simulink model "ModelEnv_Test_Erreur_tracker_v2"  (R2020b)
settings: Solver=VariableStepAuto  StartTime=0.0  StopTime=24  RelTol=1e-3
undefined symbols (not defined in the file): alpha, Atz, Bd, Bh, gama, theta, Ts, Tz_init
libraries: dspsrcs4 x2
settings Model: Creator=masdoua1  LastModifiedBy=masdoua1

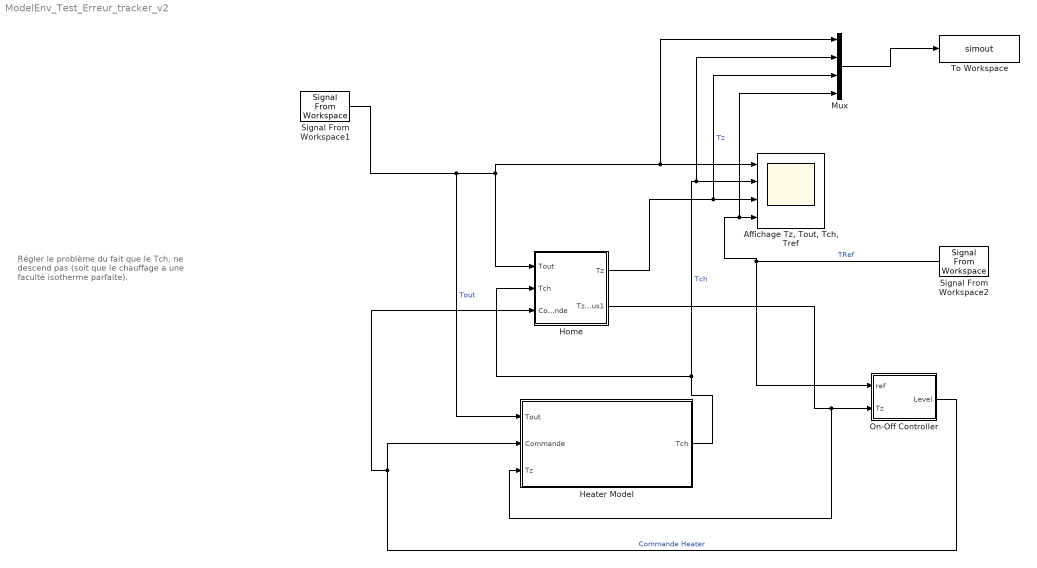
== system ModelEnv_Test_Erreur_tracker_v2 ==
  note: Régler le problème du fait que le Tch, ne descend pas (soit que le chauffage a une faculté isotherme parfaite).
  "Affichage Tz, Tout, Tch, Tref" : Scope  NumInputPorts=4
  Heater Model : Subsystem
  Home : Subsystem
  Mux : Mux
      settings: DisplayOption=signals
  On-Off Controller : MATLAB Function  TreatAsAtomicUnit=on
  Signal From Workspace1 : dspsrcs4/Signal From Workspace  X=Tout  Ts=1  nsamps=1  OutputAfterFinalValue=Setting to zero  ignoreOrWarnInputAndFrameLengths=off  OutputFrames=off
  Signal From Workspace2 : dspsrcs4/Signal From Workspace  X=Ref  Ts=1  nsamps=1  OutputAfterFinalValue=Setting to zero  ignoreOrWarnInputAndFrameLengths=off  OutputFrames=off
  To Workspace : ToWorkspace  VariableName=simout  SaveFormat=Timeseries  SampleTime=-1
  wires:
  On-Off Controller/1(Level) -> Heater Model/2(Commande), Home/3(Commande)  "Commande Heater"
  Signal From Workspace2/1 -> On-Off Controller/1(ref), Mux/4, "Affichage Tz, Tout, Tch, Tref"/4  "TRef"
  Heater Model/1(Tch) -> Mux/2, "Affichage Tz, Tout, Tch, Tref"/2, Home/2(Tch)  "Tch"
  Signal From Workspace1/1 -> Heater Model/1(Tout), Home/1(Tout), Mux/1, "Affichage Tz, Tout, Tch, Tref"/1  "Tout"
  Home/2(Tz_minus1) -> Heater Model/3(Tz), On-Off Controller/2(Tz)
  Home/1(Tz) -> Mux/3, "Affichage Tz, Tout, Tch, Tref"/3  "Tz"
  Mux/1 -> To Workspace/1

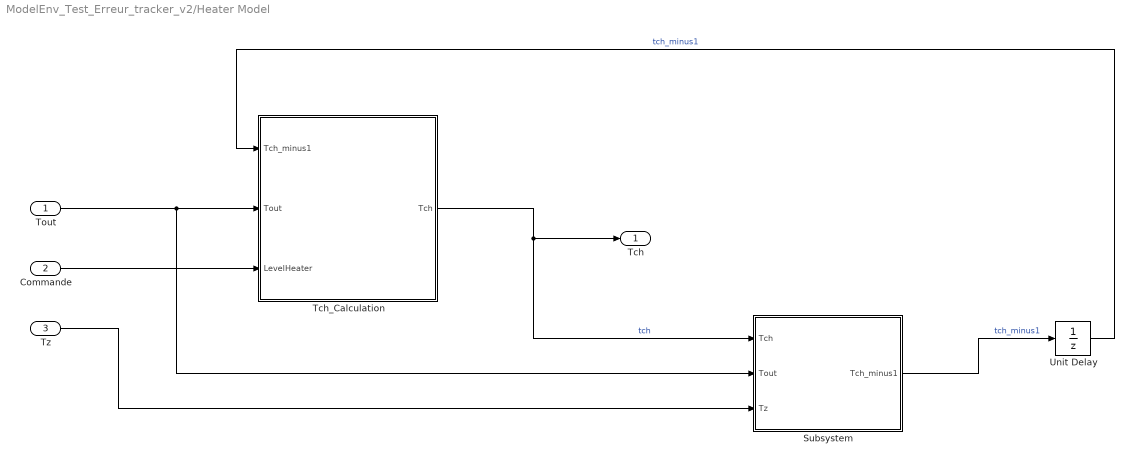
== system ModelEnv_Test_Erreur_tracker_v2/Heater Model ==
  Tout : Inport
  Commande : Inport  Port=2
  Tz : Inport  Port=3
  Subsystem : Subsystem
  Tch_Calculation : MATLAB Function  TreatAsAtomicUnit=on
  Unit Delay : UnitDelay  SampleTime=-1  HasFrameUpgradeWarning=on
  Tch : Outport
  wires:
  Tout/1 -> Subsystem/2(Tout), Tch_Calculation/2(Tout)
  Commande/1 -> Tch_Calculation/3(LevelHeater)
  Tch_Calculation/1(Tch) -> Subsystem/1(Tch), Tch/1  "tch"
  Unit Delay/1 -> Tch_Calculation/1(Tch_minus1)  "tch_minus1"
  Tz/1 -> Subsystem/3(Tz)
  Subsystem/1(Tch_minus1) -> Unit Delay/1  "tch_minus1"

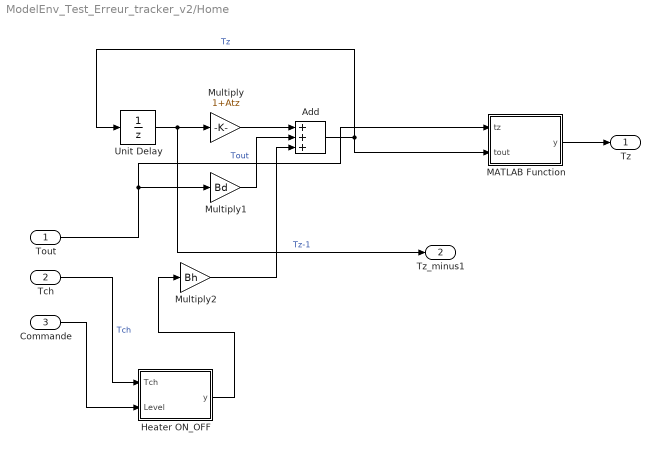
== system ModelEnv_Test_Erreur_tracker_v2/Home ==
  Tout : Inport
  Tch : Inport  Port=2
  Commande : Inport  Port=3
  Add : Sum  Inputs=+++
  Heater ON_OFF : MATLAB Function  TreatAsAtomicUnit=on
  MATLAB Function : MATLAB Function  TreatAsAtomicUnit=on
  Multiply : Gain  Gain=1+Atz
  Multiply1 : Gain  Gain=Bd
  Multiply2 : Gain  Gain=Bh
  Unit Delay : UnitDelay  InitialCondition=Tz_init  SampleTime=Ts  HasFrameUpgradeWarning=on
  Tz : Outport
  Tz_minus1 : Outport  Port=2
  wires:
  Multiply/1 -> Add/1
  Unit Delay/1 -> Tz_minus1/1, Multiply/1  "Tz-1"
  Tout/1 -> MATLAB Function/1(tz), Multiply1/1  "Tout"
  Multiply1/1 -> Add/2
  Add/1 -> Unit Delay/1, MATLAB Function/2(tout)  "Tz"
  Multiply2/1 -> Add/3
  Commande/1 -> Heater ON_OFF/2(Level)
  Tch/1 -> Heater ON_OFF/1(Tch)  "Tch"
  Heater ON_OFF/1(y) -> Multiply2/1
  MATLAB Function/1(y) -> Tz/1

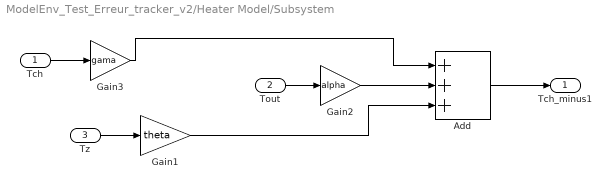
== system ModelEnv_Test_Erreur_tracker_v2/Heater Model/Subsystem ==
  Tch : Inport
  Tout : Inport  Port=2
  Tz : Inport  Port=3
  Add : Sum  Inputs=+++
  Gain1 : Gain  Gain=theta
  Gain2 : Gain  Gain=alpha
  Gain3 : Gain  Gain=gama
  Tch_minus1 : Outport
  wires:
  Add/1 -> Tch_minus1/1
  Gain1/1 -> Add/3
  Tz/1 -> Gain1/1
  Tout/1 -> Gain2/1
  Gain2/1 -> Add/2
  Tch/1 -> Gain3/1
  Gain3/1 -> Add/1

== matlab function ModelEnv_Test_Erreur_tracker_v2/Heater Model/Tch_Calculation ==
  data: Tch_minus1 input; Tout input; LevelHeater input; Tch output
function Tch = fcn(Tch_minus1, Tout, LevelHeater)
    
    if Tout > Tch_minus1
        Tch_minus1 = Tout+0.2; 
    end
    
    Tch = Tch_minus1 + LevelHeater;

== matlab function ModelEnv_Test_Erreur_tracker_v2/On-Off Controller ==
  data: ref input; Tz input; Level output
function Level= fcn(ref, Tz)

err = ref - Tz;
if err > 0
    Level = 5;
else
    Level = 0;
end
    
end

== matlab function ModelEnv_Test_Erreur_tracker_v2/Home/Heater ON_OFF ==
  data: Tch input; Level input; y output
function y = fcn(Tch, Level)
y = Tch;
if Level ==0
        y = 0;
end

== matlab function ModelEnv_Test_Erreur_tracker_v2/Home/MATLAB Function ==
  data: tz input; tout input; y output
function y = fcn(tz, tout)
y = tz;
    if tz < tout
        y = tout;
    end
